simulink model "sliding_mode_control"  (R2024b)
settings: Solver=VariableStepAuto  StartTime=0.0  StopTime=10.0  RelTol=1e-3
undefined symbols (not defined in the file or in its folder): l, m
libraries: simulink x1
settings Model: Creator=Austinchao  LastModifiedBy=Austinchao

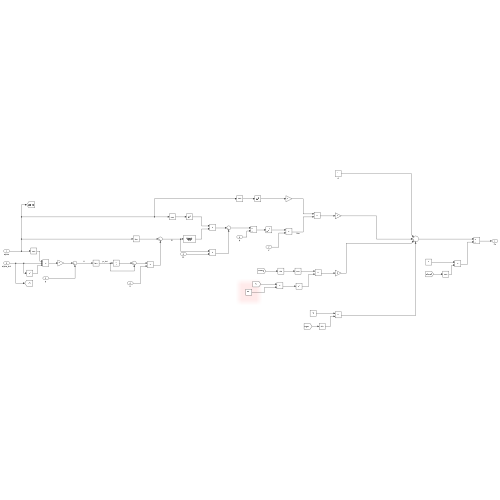
[thumbnail: Simulink's stored preview of the top-level diagram]
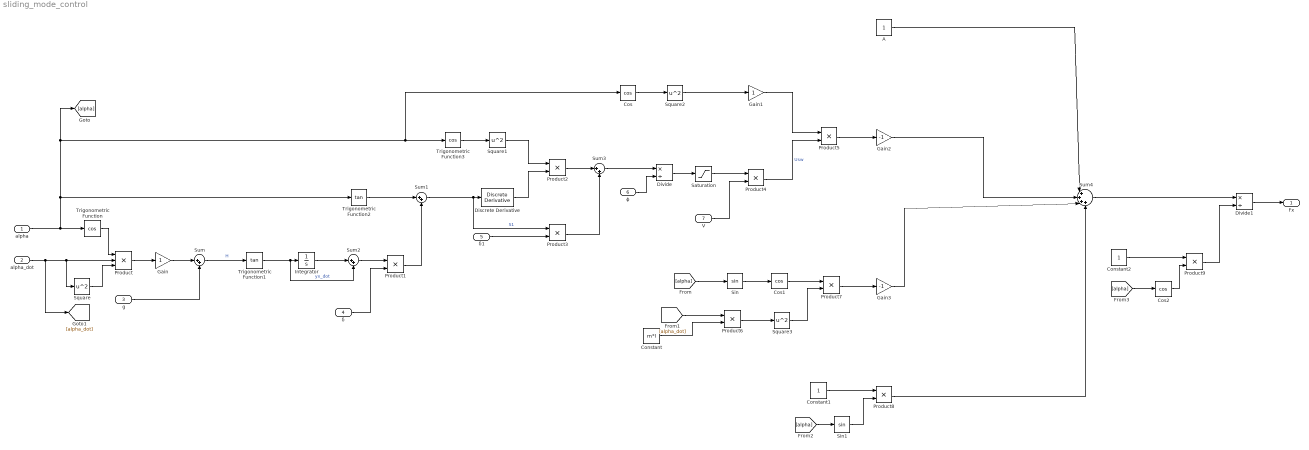
== system sliding_mode_control ==
  alpha : Inport
  alpha_dot : Inport  Port=2
  g : Inport  Port=3
  δ : Inport  Port=4
  δ1 : Inport  Port=5
  ϕ : Inport  Port=6
  V : Inport  Port=7
  A : Constant
  Constant : Constant  Value=m*l
  Constant1 : Constant
  Constant2 : Constant
  Cos : Trigonometry  Operator=cos
  Cos1 : Trigonometry  Operator=cos
  Cos2 : Trigonometry  Operator=cos
  Discrete Derivative : simulink/Discrete/Discrete Derivative  gainval=1.0  ICPrevScaledInput=0.0  OutMin=[]  OutMax=[]  OutDataType=fixdt(1, 16)  OutScaling=2^-10  DoSatur=off
  Divide : Product  Inputs=*/
  Divide1 : Product  Inputs=*/
  Gain : Gain
  Gain1 : Gain
  Gain2 : Gain  Gain=-1
  Gain3 : Gain  Gain=-1
  Integrator : Integrator
  Product : Product  Inputs=3
  Product{1..9} (9 alike) : Product
  Saturation : Saturate  UpperLimit=1  LowerLimit=-1
  Sin : Trigonometry
  Sin1 : Trigonometry
  Square{,1..3} (4 alike) : Math  Operator=square
  Sum{,1..3} (4 alike) : Sum  Inputs=|++
  Sum4 : Sum  Inputs=|++++
  Trigonometric Function : Trigonometry  Operator=cos
  Trigonometric Function1 : Trigonometry  Operator=tan
  Trigonometric Function2 : Trigonometry  Operator=tan
  Trigonometric Function3 : Trigonometry  Operator=cos
  Fx : Outport
  wires:
  alpha/1 -> Trigonometric Function2/1, [alpha], Cos/1, Trigonometric Function3/1, Trigonometric Function/1
  g/1 -> Sum/2
  alpha_dot/1 -> [alpha_dot], Product/2, Square/1
  Trigonometric Function/1 -> Product/1
  Product/1 -> Gain/1
  Gain/1 -> Sum/1
  Sum/1 -> Trigonometric Function1/1  "H"
  Trigonometric Function1/1 -> Sum2/2, Integrator/1  "yx_dot"
  Trigonometric Function2/1 -> Sum1/1
  Integrator/1 -> Sum2/1
  Sum2/1 -> Product1/1
  δ/1 -> Product1/2
  Product1/1 -> Sum1/2
  Sum1/1 -> Product3/1, Discrete Derivative/1  "S1"
  Square/1 -> Product/3
  Square1/1 -> Product2/1
  Discrete Derivative/1 -> Product2/2
  δ1/1 -> Product3/2
  Product2/1 -> Sum3/1
  Product3/1 -> Sum3/2
  Sum3/1 -> Divide/1
  Trigonometric Function3/1 -> Square1/1
  ϕ/1 -> Divide/2
  Divide/1 -> Saturation/1
  Saturation/1 -> Product4/1
  V/1 -> Product4/2
  Cos/1 -> Square2/1
  Square2/1 -> Gain1/1
  Gain1/1 -> Product5/1
  Product4/1 -> Product5/2  "Usw"
  Product5/1 -> Gain2/1
  Constant/1 -> Product6/2
  Product6/1 -> Square3/1
  [alpha] -> Sin/1
  Sin/1 -> Cos1/1
  Cos1/1 -> Product7/1
  Square3/1 -> Product7/2
  Product7/1 -> Gain3/1
  [alpha_dot] -> Product6/1
  Constant1/1 -> Product8/1
  [alpha] -> Sin1/1
  Sin1/1 -> Product8/2
  A/1 -> Sum4/1
  Gain2/1 -> Sum4/2
  Gain3/1 -> Sum4/3
  Product8/1 -> Sum4/4
  Sum4/1 -> Divide1/1
  [alpha] -> Cos2/1
  Divide1/1 -> Fx/1
  Constant2/1 -> Product9/1
  Cos2/1 -> Product9/2
  Product9/1 -> Divide1/2
